simulink model "REMUS_Glider"  (R2019b)
settings: Solver=VariableStepAuto  StartTime=0.0  StopTime=70  RelTol=1e-3
settings Model: Creator=7385281  LastModifiedBy=7385281
settings DataIOCC: SaveOutput=off  ReturnWorkspaceOutputs=off

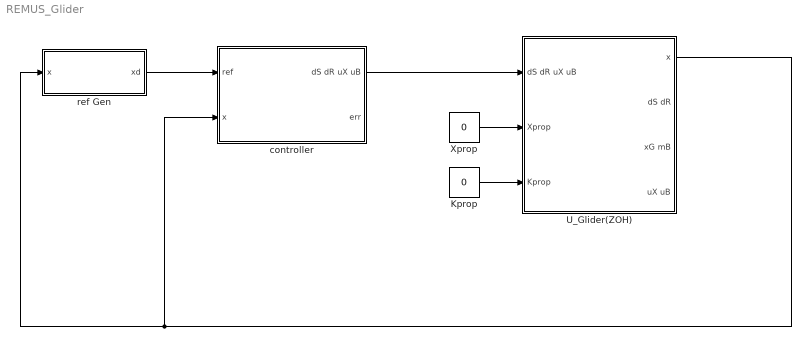
== system REMUS_Glider ==
  Kprop : Constant  Value=0
  U_Glider(ZOH) : Subsystem
  Xprop : Constant  Value=0
  controller : Subsystem
  ref Gen : Subsystem
  wires:
  Xprop/1 -> U_Glider(ZOH)/2(Xprop)
  Kprop/1 -> U_Glider(ZOH)/3(Kprop)
  controller/1(dS dR uX uB) -> U_Glider(ZOH)/1(dS dR uX uB)
  ref Gen/1(xd) -> controller/1(ref)
  U_Glider(ZOH)/1(x) -> controller/2(x), ref Gen/1(x)

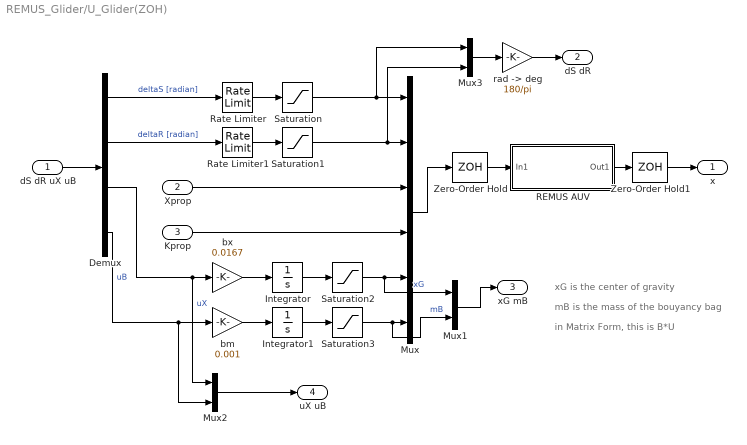
== system REMUS_Glider/U_Glider(ZOH) ==
  note: in Matrix Form, this is B*U
  note: mB is the mass of the bouyancy bag
  note: xG is the center of gravity
  dS dR uX uB : Inport
  Xprop : Inport  Port=2
  Kprop : Inport  Port=3
  Demux : Demux
  Integrator : Integrator
  Integrator1 : Integrator
  Mux : Mux  Inputs=6
  Mux1 : Mux  Inputs=2
  Mux2 : Mux  Inputs=2
  Mux3 : Mux  Inputs=2
  REMUS AUV : Subsystem
  Rate Limiter : RateLimiter  SampleTimeMode=inherited
  Rate Limiter1 : RateLimiter  SampleTimeMode=inherited
  Saturation{,1..3} (4 alike) : Saturate
  Zero-Order Hold : ZeroOrderHold
  Zero-Order Hold1 : ZeroOrderHold
  bm : Gain  Gain=0.001
  bx : Gain  Gain=0.0167
  "rad -> deg" : Gain  Gain=180/pi
  x : Outport
  dS dR : Outport  Port=2
  xG mB : Outport  Port=3
  uX uB : Outport  Port=4
  wires:
  dS dR uX uB/1 -> Demux/1
  Demux/1 -> Rate Limiter/1  "deltaS [radian]"
  Rate Limiter/1 -> Saturation/1
  Demux/2 -> Rate Limiter1/1  "deltaR [radian]"
  Rate Limiter1/1 -> Saturation1/1
  Demux/3 -> Mux2/1, bx/1  "uX"
  Demux/4 -> Mux2/2, bm/1  "uB"
  Saturation/1 -> Mux3/1, Mux/1
  bx/1 -> Integrator/1
  bm/1 -> Integrator1/1
  Integrator/1 -> Saturation2/1
  Integrator1/1 -> Saturation3/1
  Saturation1/1 -> Mux3/2, Mux/2
  Mux/1 -> Zero-Order Hold/1
  Zero-Order Hold1/1 -> x/1
  Mux1/1 -> xG mB/1
  Mux2/1 -> uX uB/1
  Mux3/1 -> "rad -> deg"/1
  "rad -> deg"/1 -> dS dR/1
  Saturation3/1 -> Mux1/2, Mux/6  "mB"
  Saturation2/1 -> Mux1/1, Mux/5  "xG"
  Kprop/1 -> Mux/4
  Xprop/1 -> Mux/3
  Zero-Order Hold/1 -> REMUS AUV/1(In1)
  REMUS AUV/1(Out1) -> Zero-Order Hold1/1

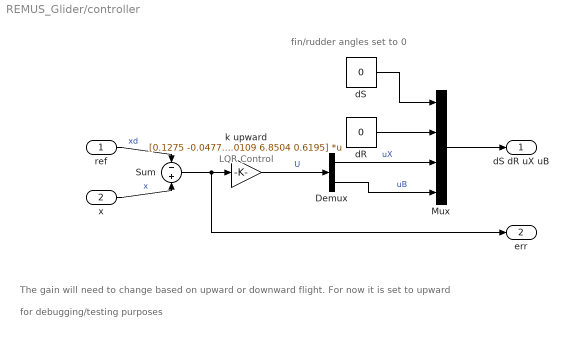
== system REMUS_Glider/controller ==
  note: LQR Control
  note: fin/rudder angles set to 0
  note: for debugging/testing purposes
  note: The gain will need to change based on upward or downward flight. For now it is set to upward
  ref : Inport
  x : Inport  Port=2
  Demux : Demux  Outputs=2
  Mux : Mux
  Sum : Sum  Inputs=-+
  dR : Constant  Value=0
  dS : Constant  Value=0
  k upward : Gain  Gain=[0.1275 -0.0477 -0.0021 -0.0009 0.0253 18.2666 0.4104; -0.0683 -0.0196 -0.0049 -0.0004 0.0109 6.8504 0.6195]  Multiplication=Matrix(K*u)
  dS dR uX uB : Outport
  err : Outport  Port=2
  wires:
  ref/1 -> Sum/1  "xd"
  x/1 -> Sum/2  "x"
  Sum/1 -> err/1, k upward/1
  k upward/1 -> Demux/1  "U"
  Demux/1 -> Mux/3  "uX"
  Demux/2 -> Mux/4  "uB"
  dS/1 -> Mux/1
  dR/1 -> Mux/2
  Mux/1 -> dS dR uX uB/1

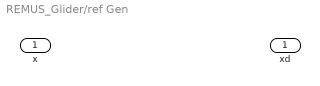
== system REMUS_Glider/ref Gen ==
  x : Inport
  xd : Outport

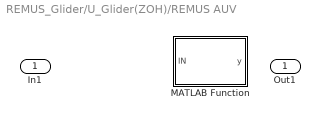
== system REMUS_Glider/U_Glider(ZOH)/REMUS AUV ==
  In1 : Inport
  MATLAB Function : MATLAB Function  TreatAsAtomicUnit=on
  Out1 : Outport

== matlab function REMUS_Glider/U_Glider(ZOH)/REMUS AUV/MATLAB Function ==
  data: IN input; y output
function y = fcn(IN)
%--------------------------------------------------------------------------
% AUV Parameter Constants [units: Metric]:
mh = 30.4791;
mbar = 1;
m = 32.3140;
g = 9.81;

xb = 0;
yb = 0;
zb = 0;
xg = 0;
yg = 0;
zg = 0.02;

Ixx = 0.177;
Iyy = 3.45;
Izz = 3.45;

Xudot = -0.93; 
Zwdot = -35.5;
Zqdot = -1.93;
Yvdot = -35.5;
Yrdot = 1.93;
Xuu = -3.9;

Yvv = -1310;
Yrr = 0.632;
Yuv = -18.96;
Yuudr = 9.64;
Yuvf = -9.64;
Yurf = 6.15;

Zww = -131;
Zqq = -0.6320;
Zuw = -18.96;
Zuuds = -9.64;
Zuwf = -9.64;
Zuqa = 0.93;
Zuqf = -6.15;

Kpdot = -0.0704;
Kpp = -0.13;

Mwdot = -1.93;
Mqdot = -4.88;
Mww = 3.18;
Mqq = -188;
Muw = -4.42;
Muuds = -6.15;
Muwf = -6.15;
Muqf = -3.93;

Nvdot =1.93;
Nrdot = -4.88;
Nvv = -3.18;
Nrr = -94;
Nuv = 4.45;
Nuudr = -6.15;
Nuvf = 6.15;
Nurf = -3.93;
%--------------------------------------------------------------------------

%--------------------------------------------------------------------------
% % INPUT PARAMETERS:
dS = IN(1);
dR = IN(2);
Xprop = IN(3);
Kprop = IN(4);
xG = IN(5);
mB = IN(6);
%--------------------------------------------------------------------------

%--------------------------------------------------------------------------
% Calculated Terms:

y = u;
